simulink model "PI controller to simulate ev3 mobile robot dynamics"  (R2021a)
settings: Solver=VariableStepAuto  StartTime=0.0  StopTime=10  RelTol=1e-3
settings Model: Creator=sanch  LastModifiedBy=hritw
settings SolverCC: AlgebraicLoopSolver=TrustRegion
settings DebuggingCC: SFMachineParentedDataDiag=warning

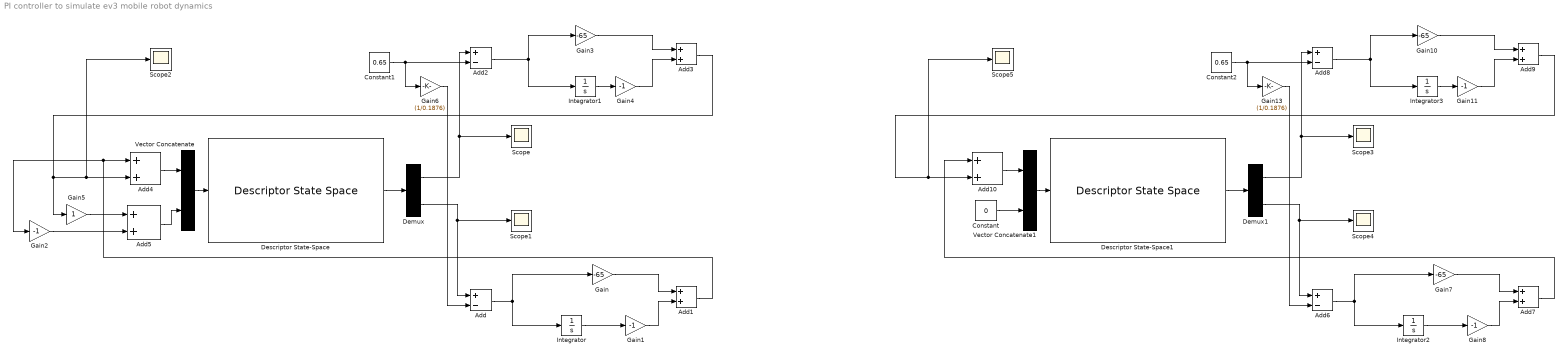
== system PI controller to simulate ev3 mobile robot dynamics ==
  Add{,2,6,8} (4 alike) : Sum  Inputs=+-
  Add{1,3..5,7,9..10} (7 alike) : Sum
  Constant : Constant  Value=0
  Constant1 : Constant  Value=0.65
  Constant2 : Constant  Value=0.65
  Demux : Demux  Outputs=2
  Demux1 : Demux  Outputs=2
  Descriptor State-Space : DescriptorStateSpace  E=[1 0;0 1]  A=[-2.2422 0;0 -2.1672]  B=[.3382 .3382;1.2219 -1.2219]  C=[1 0;0 1]  D=[0 0;0 0]  InitialCondition=[0;0]
  Descriptor State-Space1 : DescriptorStateSpace  E=[1 0;0 1]  A=[-2.2422 0;0 -2.1672]  B=[.3382 .3382;1.2219 -1.2219]  C=[1 0;0 1]  D=[0 0;0 0]  InitialCondition=[0;0]
  Gain{,3,7,10} (4 alike) : Gain  Gain=-65
  Gain{1..2,4,8,11} (5 alike) : Gain  Gain=-1
  Gain13 : Gain  Gain=(1/0.1876)
  Gain5 : Gain
  Gain6 : Gain  Gain=(1/0.1876)
  Integrator{,1..3} (4 alike) : Integrator
  Scope{,1..5} (6 alike) : Scope
  Vector Concatenate : Concatenate
  Vector Concatenate1 : Concatenate
  wires:
  Vector Concatenate/1 -> Descriptor State-Space/1
  Descriptor State-Space/1 -> Demux/1
  Add1/1 -> Gain2/1, Add4/1
  Gain2/1 -> Add5/2
  Demux/2 -> Add/1, Scope1/1
  Demux/1 -> Scope/1, Add2/1
  Gain6/1 -> Add/2
  Add/1 -> Gain/1, Integrator/1
  Integrator/1 -> Gain1/1
  Gain/1 -> Add1/1
  Gain1/1 -> Add1/2
  Integrator1/1 -> Gain4/1
  Gain4/1 -> Add3/2
  Gain3/1 -> Add3/1
  Constant1/1 -> Add2/2, Gain6/1
  Add2/1 -> Integrator1/1, Gain3/1
  Add5/1 -> Vector Concatenate/2
  Add4/1 -> Vector Concatenate/1
  Add3/1 -> Gain5/1, Scope2/1, Add4/2
  Gain5/1 -> Add5/1
  Gain11/1 -> Add9/2
  Add8/1 -> Integrator3/1, Gain10/1
  Add10/1 -> Vector Concatenate1/1
  Gain13/1 -> Add6/2
  Integrator3/1 -> Gain11/1
  Constant/1 -> Vector Concatenate1/2
  Constant2/1 -> Add8/2, Gain13/1
  Vector Concatenate1/1 -> Descriptor State-Space1/1
  Add7/1 -> Add10/1
  Demux1/2 -> Add6/1, Scope4/1
  Add9/1 -> Scope5/1, Add10/2
  Demux1/1 -> Scope3/1, Add8/1
  Add6/1 -> Gain7/1, Integrator2/1
  Gain8/1 -> Add7/2
  Gain10/1 -> Add9/1
  Integrator2/1 -> Gain8/1
  Descriptor State-Space1/1 -> Demux1/1
  Gain7/1 -> Add7/1
